simulink model "MotorSim"  (R2017a)
settings: Solver=VariableStepAuto  StartTime=0.0  StopTime=10.0  RelTol=1e-3
libraries: fl_lib x7, nesl_utility x4
settings Model: Creator=mcall  LastModifiedBy=mcall

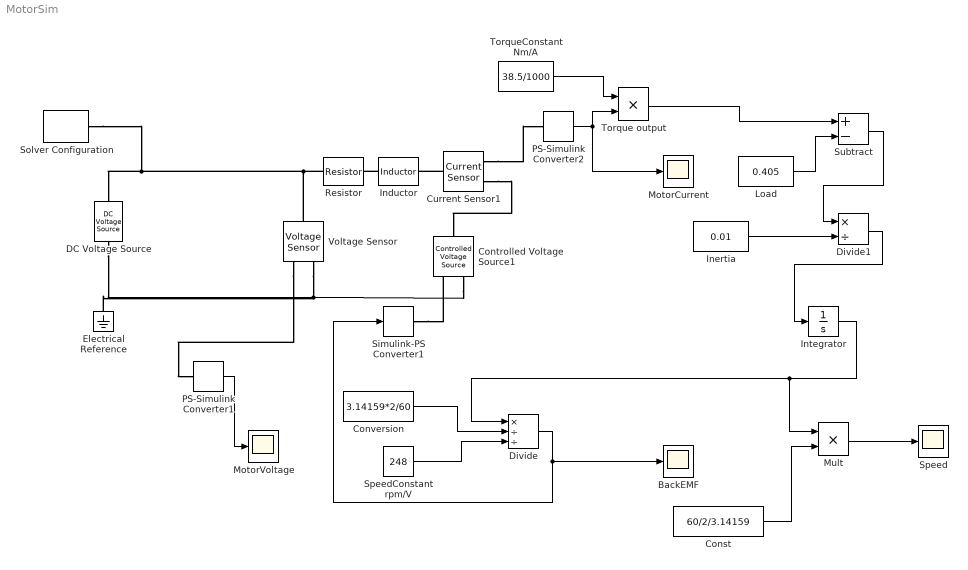
== system MotorSim ==
  BackEMF : Scope
  Const : Constant  Value=60/2/3.14159
  Controlled Voltage Source1 : fl_lib/Electrical/Electrical Sources/Controlled Voltage Source
  Conversion : Constant  Value=3.14159*2/60
  Current Sensor1 : fl_lib/Electrical/Electrical Sensors/Current Sensor
  DC Voltage Source : fl_lib/Electrical/Electrical Sources/DC Voltage Source  v0=24 V
  Divide : Product  Inputs=*//
  Divide1 : Product  Inputs=*/
  Electrical Reference : fl_lib/Electrical/Electrical Elements/Electrical Reference
  Inductor : fl_lib/Electrical/Electrical Elements/Inductor  l=0.072 mH  r=0 Ohm  g=1e-9 1/Ohm  i_specify=off  i_priority=None  i=0 A  i_nominal_specify=off  i_nominal_unit=A  i_nominal_value=1  v_specify=off  v_priority=None  v=0 V  v_nominal_specify=off  v_nominal_unit=V  v_nominal_value=1  i_L_specify=off  i_L_priority=High  i_L=0 A  i_L_nominal_specify=off  i_L_nominal_unit=A  i_L_nominal_value=1
  Inertia : Constant  Value=0.01
  Integrator : Integrator
  Load : Constant  Value=0.405
  MotorCurrent : Scope
  MotorVoltage : Scope
  Mult : Product
  PS-Simulink Converter1 : nesl_utility/PS-Simulink Converter  PhysicalDomain=network_engine_domain  SubClassName=ps_output  LeftPortType=input  RightPortType=output  PseudoPeriodic=off  Frequencies=[]  Unit=1  AffineConversion=off
  PS-Simulink Converter2 : nesl_utility/PS-Simulink Converter  PhysicalDomain=network_engine_domain  SubClassName=ps_output  LeftPortType=input  RightPortType=output  PseudoPeriodic=off  Frequencies=[]  Unit=1  AffineConversion=off
  Resistor : fl_lib/Electrical/Electrical Elements/Resistor  R=0.103 Ohm  i_specify=off  i_priority=None  i=0 A  i_nominal_specify=off  i_nominal_unit=A  i_nominal_value=1  v_specify=off  v_priority=None  v=0 V  v_nominal_specify=off  v_nominal_unit=V  v_nominal_value=1
  Simulink-PS Converter1 : nesl_utility/Simulink-PS Converter  PhysicalDomain=network_engine_domain  SubClassName=ps_input  LeftPortType=input  RightPortType=output  PseudoPeriodic=off  Frequencies=[]  NoiseDistribution=none  NoiseParameters=[]  Unit=1  AffineConversion=off  FilteringAndDerivatives=provide  SimscapeFilterOrder=1  InputFilterTimeConstant=0.001  UdotUserProvided=0
  Solver Configuration : nesl_utility/Solver Configuration  PhysicalDomain=network_engine_domain  SubClassName=solver  LeftPortType=input  RightPortType=generic  Accelerate=off  Tones=[]  Harmonics=[]  SimulateNoise=off  Profile=off  UseLocalSampling=off  EnableSwitchedLinearOptims=on  FrequencyDomain=off  UseCCode=off  RelTol=0.001  AbsTol=1e-06  MinStep=1e-09  ToWorkspace=off  RevertToSquareIcSolve=off  NumHomotopyIterations=100  PhasorMode=off  PhasorModeNumHarmonics=1  OverrideAbsTol=off  DoDC=off  ResidualTolerance=1e-09  UseLocalSolver=off  LocalSolverChoice=NE_BACKWARD_EULER_ADVANCER  LocalSolverSampleTime=0.001  DoFixedCost=off  MaxNonlinIter=3  MaxModeIter=2  LinearAlgebra=Sparse  DelaysMemoryBudget=1024  AutomaticFiltering=on  FilteringTimeConstant=0.001
  Speed : Scope
  SpeedConstant rpm/V : Constant  Value=248
  Subtract : Sum  Inputs=+-
  Torque output : Product
  TorqueConstant Nm/A : Constant  Value=38.5/1000
  Voltage Sensor : fl_lib/Electrical/Electrical Sensors/Voltage Sensor
  wires:
  PS-Simulink Converter1/1 -> MotorVoltage/1
  Divide/1 -> Simulink-PS Converter1/1, BackEMF/1
  TorqueConstant Nm/A/1 -> Torque output/1
  PS-Simulink Converter2/1 -> MotorCurrent/1, Torque output/2
  Conversion/1 -> Divide/2
  Integrator/1 -> Mult/1, Divide/1
  SpeedConstant rpm/V/1 -> Divide/3
  Inertia/1 -> Divide1/2
  Divide1/1 -> Integrator/1
  Mult/1 -> Speed/1
  Const/1 -> Mult/2
  Torque output/1 -> Subtract/1
  Load/1 -> Subtract/2
  Subtract/1 -> Divide1/1
  connections:
  Voltage Sensor/LConn1 -- Solver Configuration/RConn1 -- DC Voltage Source/LConn1 -- Resistor/LConn1
  Controlled Voltage Source1/RConn2 -- Electrical Reference/LConn1 -- DC Voltage Source/RConn1 -- Voltage Sensor/RConn2
  Current Sensor1/LConn1 -- Inductor/RConn1
  Current Sensor1/RConn2 -- Controlled Voltage Source1/LConn1
  Voltage Sensor/RConn1 -- PS-Simulink Converter1/LConn1
  Simulink-PS Converter1/RConn1 -- Controlled Voltage Source1/RConn1
  Inductor/LConn1 -- Resistor/RConn1
  Current Sensor1/RConn1 -- PS-Simulink Converter2/LConn1
